simulink model "Single_Interlinking_Dual_Infinite_Bus_Window"  (R2024b)
settings: Solver=FixedStepAuto  StartTime=0  StopTime=35  FixedStep=Ts  RelTol=1e-3
InitFcn:
  | FS_Frequency=csvread("Frequency_Sweep_Log_Matched.csv",1,0);
values from neighbouring files (symbols this model uses):
  x_e = [i_d; i_q; i_d_i; i_q_i; v_d_i; v_q_i; theta; v_dc; v_dc_i; i; i_i; v_lk; p_sum_i; p_lk_i]    [InterlinkAcDcB2B.m]
undefined symbols (not defined in the file or in its folder): ApparatusDiscreDamping, ApparatusPara, ApparatusPowerFlow, ApparatusType, OtherInputs, PowerFlow, Ts, Wbase, Ybase, Zbase
libraries: SimplusGT x8, dspindex x4, spsControlledVoltageSourceLib x3, spsGroundLib x2, spsabctodq0Lib x2, spsThreePhaseSeriesRLCBranchLib x1, spsThreePhaseParallelRLCBranchLib x1, spsParallelRLCBranchLib x1, spsThreePhaseVIMeasurementLib x1, spsdq0toabcLib x1, sps_lib x1
settings Model: Creator=gzhan  LastModifiedBy=gzhan

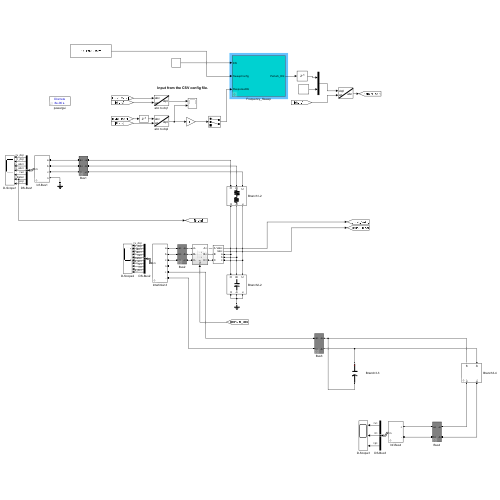
[thumbnail: Simulink's stored preview of the top-level diagram]
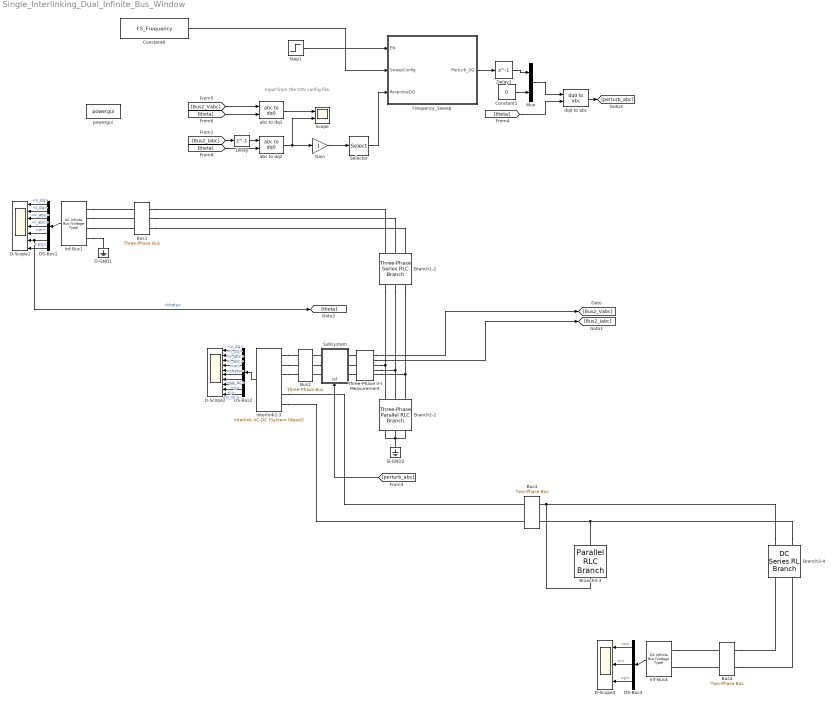
== system Single_Interlinking_Dual_Infinite_Bus_Window ==
  note: Input from the CSV config file.
  B-GND2 : spsGroundLib/Ground  LConnTagsString=a
  Branch1-2 : spsThreePhaseSeriesRLCBranchLib/Three-Phase Series RLC Branch  LConnTagsString=A|B|C  RConnTagsString=A|B|C  BranchType=RL  Resistance=(0.06)*Zbase  Inductance=(0.3)*Zbase/Wbase  Capacitance=1e-6  Measurements=None
  Branch2-2 : spsThreePhaseParallelRLCBranchLib/Three-Phase Parallel RLC Branch  LConnTagsString=A|B|C  RConnTagsString=A|B|C  BranchType=C  Resistance=(Inf)*Zbase  Inductance=(Inf)*Zbase/Wbase  Capacitance=(0.02)*Ybase/Wbase  Measurements=None
  Branch3-3 : spsParallelRLCBranchLib/Parallel RLC Branch  LConnTagsString=a  RConnTagsString=__new0  BranchType=C  Resistance=(Inf)*Zbase  Inductance=(Inf)*Zbase/Wbase  SetiL0=off  InitialCurrent=0  Capacitance=(0.02)*Ybase/Wbase  Setx0=off  InitialVoltage=0  Measurements=None
  Branch3-4 : SimplusGT/DC Series RL Branch  BranchType=RL  Resistance=(0.01)*Zbase  Inductance=(0.3)*Zbase/Wbase
      settings: SourceProductName=Simplus Grid Tool
  Bus1 : SimplusGT/Three-Phase Bus  Vbase=1  Sbase=1
      settings: SourceProductName=Simplus Grid Tool
  Bus2 : SimplusGT/Three-Phase Bus  Vbase=1  Sbase=1
      settings: SourceProductName=Simplus Grid Tool
  Bus3 : SimplusGT/Two-Phase Bus  Vbase=1  Sbase=1
      settings: SourceProductName=Simplus Grid Tool
  Bus4 : SimplusGT/Two-Phase Bus  Vbase=1  Sbase=1
      settings: SourceProductName=Simplus Grid Tool
  Constant1 : Constant  Value=0
  Constant8 : Constant  Value=FS_Frequency
  D-GND1 : spsGroundLib/Ground  LConnTagsString=a
  D-Scope1 : Scope  NumInputPorts=7
  D-Scope2 : Scope  NumInputPorts=10
  D-Scope3 : Scope  NumInputPorts=3
  DS-Bus1 : BusSelector  OutputSignals=v_dq,i_dq,v_abc,i_abc,w,theta,pq
  DS-Bus2 : BusSelector  OutputSignals=v_dq,i_dq,v_abc,i_abc,w,theta,pq_ac,v,i,p_dc
  DS-Bus3 : BusSelector  OutputSignals=v,i,p
  Delay : Delay  DelayLength=1
  Delay1 : Delay  DelayLength=1
  Frequency_Sweep : Subsystem  mask{Gain=0.1, Interval=1e-1}
      mask prompts: Gain "Output Gain"; Interval "Injection Interval"
  Gain : Gain  Gain=-1
  Inf-Bus1 : SimplusGT/AC Infinite Bus (Voltage Type)  Ts=Ts  Sbase=Sbase  Vbase=Vbase  Wbase=Wbase  vd=PowerFlow{1}(3)  vq=0  theta0=PowerFlow{1}(4)  w=Wbase  R=1e-30
      settings: SourceProductName=Simplus Grid Tool
  Inf-Bus4 : SimplusGT/DC Infinite Bus (Voltage Type)  Ts=Ts  Sbase=Sbase  Vbase=Vbase  v=PowerFlow{3}(3)  R=1e-30
      settings: SourceProductName=Simplus Grid Tool
  Interlink2-3 : SimplusGT/Interlink AC-DC (System Object)  Ts=Ts  Sbase=Sbase  Vbase=Vbase  Wbase=Wbase  ApparatusType=ApparatusType{2}  ApparatusPara=ApparatusPara{2}  PowerFlow=ApparatusPowerFlow{2}  x0=x_e{2}  OtherInputs=OtherInputs{2}  DiscreMethod=Hybrid Trapezoidal  EnableInsideModification=off  DiscreDampingFlag=on  DiscreDampingValue=ApparatusDiscreDamping{2}  LinearizationTimes=1  DirectFeedthrough=off
      settings: SourceProductName=Simplus Grid Tool
  Mux : Mux  Inputs=2
  Scope : Scope  NumInputPorts=2
  Selector : Selector  InputPortWidth=3  IndexOptions=Index vector (dialog)  Indices=[1 2]  OutputSizes=1
  Step1 : Step  Time=5  SampleTime=0
  Subsystem : Subsystem
      settings: PortSchema="{\"entries\":[{\"content\":{\"sides\":[{\"content\":{\"connectorIds\":[\"LConn1\",\"LConn2\",\"LConn3\"]},\"type\":\"ConnectorPlacement.EquallySpacedRectSide\",\"uuid\":\"320e3ad3-fe57-42ad-8679-028db54dd479\"},{\"content\":{\"connectorIds\":[\"RConn1\",\"RConn2\",\"RConn3\"],\"side\":\"RIGHT\"},\"type\":\"ConnectorPlacement.EquallySpacedRectSide\",\"uuid\":\"2b28e415-5225-4c3e-a28b-d8614ba274c6\"},{\"content\":{\"side\":\"TOP\"},\"type\":\"ConnectorPlacement.EquallySpacedRectSide\",\"uuid\":\"80974e19-6780-437b-9c92-3d578e35f276\"},{\"content\":{\"connectorIds\":[\"In1\"],\"side\":\"BOTTOM\"},\"type\":\"ConnectorPlacement.EquallySpacedRectSide\",\"uuid\":\"7f793f19-b02b-48c7-b373-3f4568a43fb5\"}]},\"type\":\"ConnectorPlacement.EquallySpacedConnector\",\"uuid\":\"fbbab89f-d0d6-4a2b-bd71-75cb5c2a328e\"}],\"packageUris\":[\"http://schema.mathworks.com/mf0/Connector/R2020b\"],\"version\":\"1.0\"}"
  Three-Phase V-I Measurement : spsThreePhaseVIMeasurementLib/Three-Phase V-I Measurement  VoltageMeasurement=phase-to-ground  SetLabelV=off  LabelV=Vabc  Vpu=off  VpuLL=off  CurrentMeasurement=yes  SetLabelI=off  LabelI=Iabc  Ipu=off  Pbase=100e6  Vbase=500e3  OutputType=Complex  PhasorSimulation=off  PSBequivalent=0
  abc to dq1 : spsabctodq0Lib/abc to dq0  Alignment=90 degrees behind phase A axis
  abc to dq2 : spsabctodq0Lib/abc to dq0  Alignment=90 degrees behind phase A axis
  dq0 to abc : spsdq0toabcLib/dq0 to abc  Alignment=90 degrees behind phase A axis
  powergui : sps_lib/powergui  Priority=1  SimulationMode=Discrete  SampleTime=Ts  frequency=60  Iterations=50  frequencyindice=0  Pbase=100e6  ErrMax=1e-4  UnitsV=kV  UnitsW=MW  buscounter=0  FunctionMessages=off  echomessages=off  EnableUseOfTLC=off  CurrentSourceSwitches=off  DisableSnubberDevices=off  DisableRonSwitches=off  DisableVfSwitches=off  DisplayEquations=off  AutomaticDiscreteSolvers=off  SolverType=Tustin/Backward Euler (TBE)  Interpol=off  ExternalGateDelay=off  methode=off  Ts=100  x0status=blocks  SPID=on  SwTol=0  HookPort=off  NonlinearTolerance=1e-4  nMaxIteration=100  ContinueOnMaxIteration=off  RestoreLinks=warning  ResistiveCurrentMeasurement=off  Frange=[0:2:500]  Ylog=off  Xlog=on  ShowGrid=off  save=off  variable=ZData  structure=0  ZoomFFT=off  StartTime=0.0  cycles=1  DisplayStyle=1  fundamental=60  FreqAxis=off  MaxFrequency=1000  frequencyindicesteady=1  RmsSteady=1  display=off
  wires:
  Inf-Bus1/1 -> DS-Bus1/1
  DS-Bus1/1 -> D-Scope1/1  "<v_dq>"
  DS-Bus1/2 -> D-Scope1/2  "<i_dq>"
  DS-Bus1/3 -> D-Scope1/3  "<v_abc>"
  DS-Bus1/4 -> D-Scope1/4  "<i_abc>"
  DS-Bus1/5 -> D-Scope1/5  "<w>"
  DS-Bus1/6 -> [theta], D-Scope1/6  "<theta>"
  DS-Bus1/7 -> D-Scope1/7  "<pq>"
  DS-Bus2/1 -> D-Scope2/1  "<v_dq>"
  DS-Bus2/2 -> D-Scope2/2  "<i_dq>"
  DS-Bus2/3 -> D-Scope2/3  "<v_abc>"
  DS-Bus2/4 -> D-Scope2/4  "<i_abc>"
  DS-Bus2/5 -> D-Scope2/5  "<w>"
  DS-Bus2/6 -> D-Scope2/6  "<theta>"
  DS-Bus2/7 -> D-Scope2/7  "<pq_ac>"
  DS-Bus2/8 -> D-Scope2/8  "<v>"
  DS-Bus2/9 -> D-Scope2/9  "<i>"
  DS-Bus2/10 -> D-Scope2/10  "<p_dc>"
  Inf-Bus4/1 -> DS-Bus3/1
  DS-Bus3/1 -> D-Scope3/1  "<v>"
  DS-Bus3/2 -> D-Scope3/2  "<i>"
  DS-Bus3/3 -> D-Scope3/3  "<p>"
  abc to dq1/1 -> Scope/1
  [theta] -> abc to dq1/2
  [Bus2_Iabc] -> Delay/1
  Gain/1 -> Selector/1
  Mux/1 -> dq0 to abc/1
  Step1/1 -> Frequency_Sweep/1(EN)
  [theta] -> abc to dq2/2
  Constant1/1 -> Mux/2
  [Bus2_Vabc] -> abc to dq1/1
  Delay/1 -> abc to dq2/1
  [theta] -> dq0 to abc/2
  Delay1/1 -> Mux/1
  abc to dq2/1 -> Scope/2, Gain/1
  Selector/1 -> Frequency_Sweep/3(ResponseDQ)
  Frequency_Sweep/1(Perturb_DQ) -> Delay1/1
  Constant8/1 -> Frequency_Sweep/2(SweepConfig)
  dq0 to abc/1 -> [perturb_abc]
  Three-Phase V-I Measurement/1 -> [Bus2_Vabc]
  [perturb_abc] -> Subsystem/1(ref)
  Three-Phase V-I Measurement/2 -> [Bus2_Iabc]
  Interlink2-3/1 -> DS-Bus2/1
  connections:
  Inf-Bus1/LConn4 -- D-GND1/LConn1
  Branch2-2/RConn1 -- Branch2-2/RConn2 -- Branch2-2/RConn3 -- B-GND2/LConn1
  Branch1-2/RConn1 -- Three-Phase V-I Measurement/RConn1 -- Branch2-2/LConn1
  Branch1-2/RConn2 -- Three-Phase V-I Measurement/RConn2 -- Branch2-2/LConn2
  Branch1-2/RConn3 -- Three-Phase V-I Measurement/RConn3 -- Branch2-2/LConn3
  Bus1/RConn1 -- Branch1-2/LConn1
  Bus1/RConn2 -- Branch1-2/LConn2
  Bus1/RConn3 -- Branch1-2/LConn3
  Bus4/RConn1 -- Branch3-4/RConn1
  Bus4/RConn2 -- Branch3-4/RConn2
  Branch3-4/LConn1 -- Bus3/RConn1 -- Branch3-3/RConn1
  Branch3-4/LConn2 -- Bus3/RConn2 -- Branch3-3/LConn1
  Inf-Bus1/LConn1 -- Bus1/LConn1
  Inf-Bus1/LConn2 -- Bus1/LConn2
  Inf-Bus1/LConn3 -- Bus1/LConn3
  Interlink2-3/LConn1 -- Bus2/LConn1
  Interlink2-3/LConn2 -- Bus2/LConn2
  Interlink2-3/LConn3 -- Bus2/LConn3
  Interlink2-3/LConn5 -- Bus3/LConn1
  Interlink2-3/LConn6 -- Bus3/LConn2
  Inf-Bus4/LConn1 -- Bus4/LConn1
  Inf-Bus4/LConn2 -- Bus4/LConn2
  Subsystem/LConn1 -- Bus2/RConn1
  Bus2/RConn2 -- Subsystem/LConn2
  Subsystem/LConn3 -- Bus2/RConn3
  Subsystem/RConn1 -- Three-Phase V-I Measurement/LConn1
  Three-Phase V-I Measurement/LConn2 -- Subsystem/RConn2
  Subsystem/RConn3 -- Three-Phase V-I Measurement/LConn3

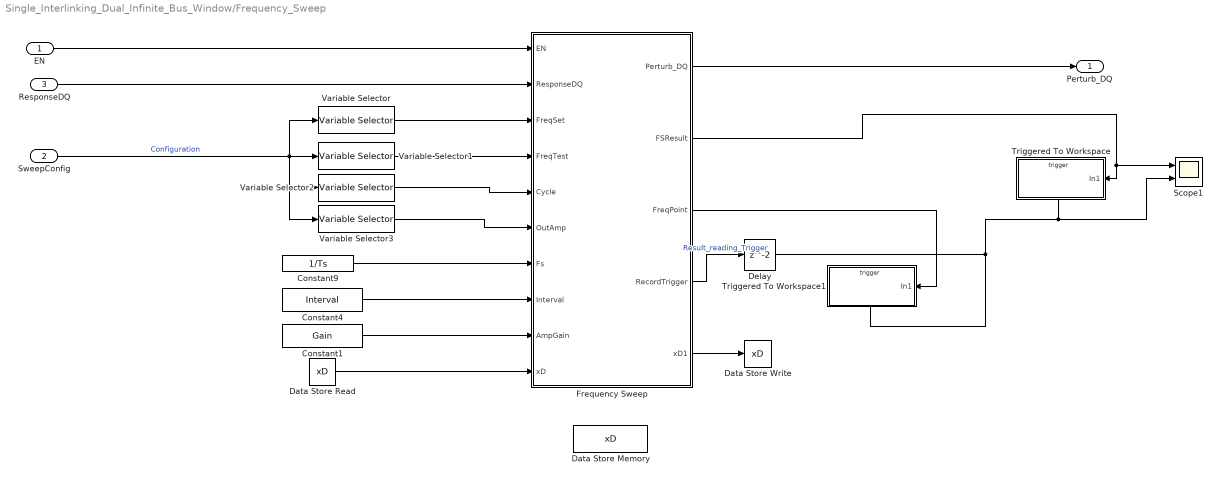
== system Single_Interlinking_Dual_Infinite_Bus_Window/Frequency_Sweep ==
  EN : Inport
  SweepConfig : Inport  Port=2
  ResponseDQ : Inport  Port=3
  Constant1 : Constant  Value=Gain
  Constant4 : Constant  Value=Interval
  Constant9 : Constant  Value=1/Ts
  Data Store Memory : DataStoreMemory  DataStoreName=xD  WriteAfterWriteMsg=warning  InitialValue=zeros(1,18)  ShowAdditionalParam=off
  Data Store Read : DataStoreRead  DataStoreName=xD  IndexOptions=Index vector (dialog)  Indices=1  OutputSizes=1
  Data Store Write : DataStoreWrite  DataStoreName=xD  IndexOptions=Index vector (dialog)  Indices=1  OutputSizes=1
  Delay : Delay
  Frequency Sweep : MATLAB Function  TreatAsAtomicUnit=on
  Scope1 : Scope  NumInputPorts=2
  Triggered To Workspace : Subsystem  AncestorBlock=dspsnks4/Triggered To Workspace  TreatAsAtomicUnit=on  mask(Triggered To Workspace){TriggerType=Rising edge, VariableName=FS_Result, Buffer=5000, Decimation=1, Save2DMode=2-D array (concatenate along first dimension), FixptAsFi=off}
      mask prompts: TriggerType "dsp:TriggeredToWorkspaceBlockDialog:TriggerType_MP"; VariableName "dsp:TriggeredToWorkspaceBlockDialog:VariableName_MP"; Buffer "dsp:TriggeredToWorkspaceBlockDialog:Buffer_MP"; Decimation "dsp:TriggeredToWorkspaceBlockDialog:Decimation_MP"; Save2DMode "dsp:TriggeredToWorkspaceBlockDialog:Save2DMode_MP"; FixptAsFi "dsp:TriggeredToWorkspaceBlockDialog:FixptAsFi_MP"
      mask help: dsp:TriggeredToWorkspaceBlockDialog:TriggeredToWorkspace_MaskDesc
      mask init:
      | dspblktrigtwks('init',TriggerType);
      settings: CopyFcn=dspblkcopystw(gcbh);
      mask Help: eval('blocksethelp');
      mask TypeOptions TriggerType: dsp:TriggeredToWorkspaceBlockDialog:TriggerType_RisingEdge | dsp:TriggeredToWorkspaceBlockDialog:TriggerType_FallingEdge | dsp:TriggeredToWorkspaceBlockDialog:TriggerType_EitherEdge
      mask TypeOptions Save2DMode: dsp:TriggeredToWorkspaceBlockDialog:Save2DMode_2DArray | dsp:TriggeredToWorkspaceBlockDialog:Save2DMode_3DArray
      mask DialogControl TriggerType Prompt: Trigger type:
      mask DialogControl VariableName Prompt: Variable name:
      mask DialogControl Buffer Prompt: Maximum number of rows:
      mask DialogControl Decimation Prompt: Decimation:
      mask DialogControl Save2DMode Prompt: Save 2-D signals as:
      mask DialogControl FixptAsFi Prompt: Log fixed-point data as a fi object
      mask Display: disp(get_param(gcbh,'VariableName'))
  Triggered To Workspace1 : Subsystem  AncestorBlock=dspsnks4/Triggered To Workspace  TreatAsAtomicUnit=on  mask(Triggered To Workspace){TriggerType=Rising edge, VariableName=FS_Freq_point, Buffer=5000, Decimation=1, Save2DMode=2-D array (concatenate along first dimension), FixptAsFi=off}
      mask prompts: TriggerType "dsp:TriggeredToWorkspaceBlockDialog:TriggerType_MP"; VariableName "dsp:TriggeredToWorkspaceBlockDialog:VariableName_MP"; Buffer "dsp:TriggeredToWorkspaceBlockDialog:Buffer_MP"; Decimation "dsp:TriggeredToWorkspaceBlockDialog:Decimation_MP"; Save2DMode "dsp:TriggeredToWorkspaceBlockDialog:Save2DMode_MP"; FixptAsFi "dsp:TriggeredToWorkspaceBlockDialog:FixptAsFi_MP"
      mask help: dsp:TriggeredToWorkspaceBlockDialog:TriggeredToWorkspace_MaskDesc
      mask init:
      | dspblktrigtwks('init',TriggerType);
      settings: CopyFcn=dspblkcopystw(gcbh);
      mask Help: eval('blocksethelp');
      mask TypeOptions TriggerType: dsp:TriggeredToWorkspaceBlockDialog:TriggerType_RisingEdge | dsp:TriggeredToWorkspaceBlockDialog:TriggerType_FallingEdge | dsp:TriggeredToWorkspaceBlockDialog:TriggerType_EitherEdge
      mask TypeOptions Save2DMode: dsp:TriggeredToWorkspaceBlockDialog:Save2DMode_2DArray | dsp:TriggeredToWorkspaceBlockDialog:Save2DMode_3DArray
      mask DialogControl TriggerType Prompt: Trigger type:
      mask DialogControl VariableName Prompt: Variable name:
      mask DialogControl Buffer Prompt: Maximum number of rows:
      mask DialogControl Decimation Prompt: Decimation:
      mask DialogControl Save2DMode Prompt: Save 2-D signals as:
      mask DialogControl FixptAsFi Prompt: Log fixed-point data as a fi object
      mask Display: disp(get_param(gcbh,'VariableName'))
  Variable Selector : dspindex/Variable Selector  NumInputs=1  rowsOrCols=Columns  IdxMode=Fixed  Elements=1  ZerOneIdxMode=One-based  errmode=Clip Index  FillMode=on  FillValues=0
  Variable Selector1 : dspindex/Variable Selector  NumInputs=1  rowsOrCols=Columns  IdxMode=Fixed  Elements=2  ZerOneIdxMode=One-based  errmode=Clip Index  FillMode=on  FillValues=0
  Variable Selector2 : dspindex/Variable Selector  NumInputs=1  rowsOrCols=Columns  IdxMode=Fixed  Elements=3  ZerOneIdxMode=One-based  errmode=Clip Index  FillMode=on  FillValues=0
  Variable Selector3 : dspindex/Variable Selector  NumInputs=1  rowsOrCols=Columns  IdxMode=Fixed  Elements=4  ZerOneIdxMode=One-based  errmode=Clip Index  FillMode=on  FillValues=0
  Perturb_DQ : Outport
  wires:
  Variable Selector2/1 -> Frequency Sweep/5(Cycle)
  Frequency Sweep/2(FSResult) -> Triggered To Workspace/1(In1), Scope1/1
  Frequency Sweep/4(RecordTrigger) -> Delay/1  "Result_reading_Trigger"
  Constant4/1 -> Frequency Sweep/8(Interval)
  Frequency Sweep/5(xD1) -> Data Store Write/1
  Variable Selector3/1 -> Frequency Sweep/6(OutAmp)
  Variable Selector1/1 -> Frequency Sweep/4(FreqTest)
  SweepConfig/1 -> Variable Selector3/1, Variable Selector2/1, Variable Selector1/1, Variable Selector/1  "Configuration"
  ResponseDQ/1 -> Frequency Sweep/2(ResponseDQ)
  Variable Selector/1 -> Frequency Sweep/3(FreqSet)
  Frequency Sweep/3(FreqPoint) -> Triggered To Workspace1/1(In1)
  Data Store Read/1 -> Frequency Sweep/10(xD)
  Constant9/1 -> Frequency Sweep/7(Fs)
  Frequency Sweep/1(Perturb_DQ) -> Perturb_DQ/1
  EN/1 -> Frequency Sweep/1(EN)
  Delay/1 -> Scope1/2, Triggered To Workspace/Trigger, Triggered To Workspace1/Trigger
  Constant1/1 -> Frequency Sweep/9(AmpGain)

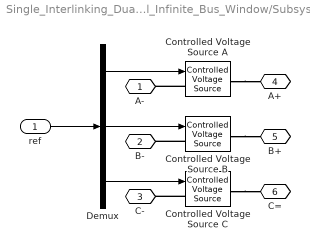
== system Single_Interlinking_Dual_Infinite_Bus_Window/Subsystem ==
  ref : Inport
  Controlled Voltage Source A : spsControlledVoltageSourceLib/Controlled Voltage Source  Initialize=on  Source_Type=AC  Amplitude=0  Phase=0  Frequency=0  Measurements=None
  Controlled Voltage Source B : spsControlledVoltageSourceLib/Controlled Voltage Source  Initialize=on  Source_Type=AC  Amplitude=0  Phase=0  Frequency=0  Measurements=None
  Controlled Voltage Source C : spsControlledVoltageSourceLib/Controlled Voltage Source  Initialize=on  Source_Type=AC  Amplitude=0  Phase=0  Frequency=0  Measurements=None
  Demux : Demux  Outputs=3
  A- : PMIOPort  Side=Left
  B- : PMIOPort  Port=2  Side=Left
  C- : PMIOPort  Port=3  Side=Left
  A+ : PMIOPort  Port=4  Side=Right
  B+ : PMIOPort  Port=5  Side=Right
  C= : PMIOPort  Port=6  Side=Right
  wires:
  Demux/3 -> Controlled Voltage Source C/1
  Demux/2 -> Controlled Voltage Source B/1
  Demux/1 -> Controlled Voltage Source A/1
  ref/1 -> Demux/1
  connections:
  Controlled Voltage Source C/RConn1 -- C=/RConn1
  Controlled Voltage Source C/LConn1 -- C-/RConn1
  Controlled Voltage Source A/LConn1 -- A-/RConn1
  Controlled Voltage Source B/LConn1 -- B-/RConn1
  Controlled Voltage Source A/RConn1 -- A+/RConn1
  Controlled Voltage Source B/RConn1 -- B+/RConn1

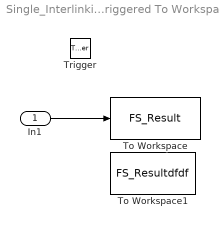
== system Single_Interlinking_Dual_Infinite_Bus_Window/Frequency_Sweep/Triggered To Workspace ==
  In1 : Inport
  Trigger : TriggerPort  VariantControl=Variant
  To Workspace : ToWorkspace  VariableName=FS_Result  SampleTime=-1
      settings: Save2DSignal=2-D array (concatenate along first dimension)
  To Workspace1 : ToWorkspace  VariableName=FS_Resultdfdf  SampleTime=-1
      settings: Save2DSignal=2-D array (concatenate along first dimension)
  wires:
  In1/1 -> To Workspace/1

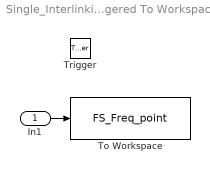
== system Single_Interlinking_Dual_Infinite_Bus_Window/Frequency_Sweep/Triggered To Workspace1 ==
  In1 : Inport
  Trigger : TriggerPort  VariantControl=Variant
  To Workspace : ToWorkspace  VariableName=FS_Freq_point  SampleTime=-1
      settings: Save2DSignal=2-D array (concatenate along first dimension)
  wires:
  In1/1 -> To Workspace/1

== matlab function Single_Interlinking_Dual_Infinite_Bus_Window/Frequency_Sweep/Frequency Sweep ==
  data: EN input; Perturb_DQ output; ResponseDQ input size=[1 2]; FreqSet input; FreqTest input; Cycle input; OutAmp input; Fs input; Interval input; AmpGain input; xD input; FSResult output; FreqPoint output; RecordTrigger output; xD1 output
function [Perturb_DQ, FSResult, FreqPoint, RecordTrigger, xD1] = fcn(EN,ResponseDQ, FreqSet, FreqTest, Cycle, OutAmp, Fs, Interval, AmpGain, xD)
% Real-time frequency scanning with Hann window + DC detrend (running mean)
%
% State variables (xD):
% xD1:  case (CaseK)
% xD2:  Ns  (total time steps for output at current frequency)
% xD3:  Nt  (total time steps for test frequency integration)
% xD4:  n   (sample count in current segment, starts at 1)
% xD5:  kc  (frequency index)
% xD6:  OutD
% xD7:  OutQ
% xD8:  SumDRe
% xD9:  SumDIm
% xD10: SumQRe
% xD11: SumQIm
% xD12: FinalDRe
% xD13: FinalDIm
% xD14: FinalQRe
% xD15: FinalQIm
% xD16: TWait
% xD17: MeanD   (running mean of ResponseDQ(1))   <-- NEW
% xD18: MeanQ   (running mean of ResponseDQ(2))   <-- NEW

% --- read states
CaseK   = xD(1);
Ns      = xD(2);
Nt      = xD(3);
n       = xD(4);
kc      = xD(5);
OutD    = xD(6);
OutQ    = xD(7);
SumDRe  = xD(8);
SumDIm  = xD(9);
SumQRe  = xD(10);
SumQIm  = xD(11);
FinalDRe= xD(12);
FinalDIm= xD(13);
FinalQRe= xD(14);
FinalQIm= xD(15);
TWait   = xD(16);
MeanD   = xD(17);   % NEW
MeanQ   = xD(18);   % NEW

FrequencyNum = length(FreqSet);

if AmpGain==0
    error('gain must not be zero');
end

%% Main Loop
if EN==0   % if Enable 0, reset just outputs (keep states unless you want full reset)
    OutD = 0;
    OutQ = 0;
else
    switch CaseK
        case 0 % the very first round
            kc    = 1;
            CaseK = 1;

        case 1 % set up D-axis sweep for this frequency index
            if kc>FrequencyNum         % sweep finished. Go to case 9
                OutD = 0;
                OutQ = 0;
                CaseK = 9;
            elseif Cycle(kc)==0        % skip this frequency
                kc = kc + 1;
            else
                % reset integrators and counters
                SumDRe = 0; SumDIm = 0; SumQRe = 0; SumQIm = 0;
                TWait  = 0; n = 0;
                MeanD  = 0; MeanQ  = 0;   % NEW: reset running means

                % total time steps for this frequency
                Ns = Fs/FreqSet(kc)*Cycle(kc); % for output count
                Nt = Fs/FreqTest(kc)*Cycle(kc); % for frequency test count

                % prime first output sample (n will become 1)
                OutD = OutAmp(kc)*sin(2*pi*Cycle(kc)*n/Ns)*AmpGain;
                OutQ = 0;
                n    = n + 1;
                CaseK= 2;
            end

        case 2 % sweep D axis: inject D, demod both D/Q responses
            OutD = OutAmp(kc)*sin(2*pi*Cycle(kc)*n/Ns)*AmpGain;
            OutQ = 0;

            % --- Hann window (periodic) at this sample (n in 1..Nt)
            w  = 0.5 - 0.5*cos(2*pi*(n-1)/Nt);

            % --- update online running means for DC detrend
            MeanD = MeanD + (ResponseDQ(1) - MeanD)/n;
            MeanQ = MeanQ + (ResponseDQ(2) - MeanQ)/n;

            % --- detrended, windowed samples
            yD = (ResponseDQ(1) - MeanD) * w;
            yQ = (ResponseDQ(2) - MeanQ) * w;

            % --- demodulate at test frequency
            sn = sin(2*pi*Cycle(kc)*(n-1)/Nt);
            cn = cos(2*pi*Cycle(kc)*(n-1)/Nt);

            % Accumulate (real=sin, imag=cos; sign convention consistent)
            SumDRe = SumDRe + yD * sn;
            SumDIm = SumDIm + yD * cn;
            SumQRe = SumQRe + yQ * sn;
            SumQIm = SumQIm + yQ * cn;

            if (n<Nt)
                n = n + 1;
            else
                OutD = 0;
                OutQ = 0;
                CaseK= 3;
            end

        case 3 % finalize D-axis phasor; wait (settling) before Q sweep
            % Hann coherent gain
            cg = 0.5;

            % Normalization (kept your original form, divided by cg)
            FinalDRe = (2*SumDRe*FreqSet(kc)/Cycle(kc)/Fs/OutAmp(kc)/AmpGain)/cg;
            FinalDIm = (2*SumDIm*FreqSet(kc)/Cycle(kc)/Fs/OutAmp(kc)/AmpGain)/cg;
            FinalQRe = (2*SumQRe*FreqSet(kc)/Cycle(kc)/Fs/OutAmp(kc)/AmpGain)/cg;
            FinalQIm = (2*SumQIm*FreqSet(kc)/Cycle(kc)/Fs/OutAmp(kc)/AmpGain)/cg;

            if TWait<Fs*Interval
                TWait = TWait + 1;
            else
                TWait = 0;
                CaseK = 4;
            end

        case 4 % prepare Q-axis sweep
            SumDRe = 0; SumDIm = 0; SumQRe = 0; SumQIm = 0;
            TWait  = 0; n = 0;
            MeanD  = 0; MeanQ  = 0;   % NEW: reset running means

            % total time steps for this frequency
            Ns = Fs/FreqSet(kc)*Cycle(kc); % for output count
            Nt = Fs/FreqTest(kc)*Cycle(kc); % for frequency test count

            OutD = 0;
            OutQ = OutAmp(kc)*sin(2*pi*Cycle(kc)*n/Ns)*AmpGain;
            n    = n + 1;
            CaseK= 5;

        case 5 % sweep Q axis: inject Q, demod both D/Q responses
            OutD = 0;
            OutQ = OutAmp(kc)*sin(2*pi*Cycle(kc)*n/Ns)*AmpGain;

            % --- Hann window (periodic)
            w  = 0.5 - 0.5*cos(2*pi*(n-1)/Nt);

            % --- running means
            MeanD = MeanD + (ResponseDQ(1) - MeanD)/n;
            MeanQ = MeanQ + (ResponseDQ(2) - MeanQ)/n;

            % --- detrended, windowed
            yD = (ResponseDQ(1) - MeanD) * w;
            yQ = (ResponseDQ(2) - MeanQ) * w;

            % --- demodulate
            sn = sin(2*pi*Cycle(kc)*(n-1)/Nt);
            cn = cos(2*pi*Cycle(kc)*(n-1)/Nt);

            % Accumulate
            SumDRe = SumDRe + yD * sn;
            SumDIm = SumDIm + yD * cn;
            SumQRe = SumQRe + yQ * sn;
            SumQIm = SumQIm + yQ * cn;

            if (n<Nt)
                n = n + 1;
            else
                OutD = 0;
                OutQ = 0;
                CaseK= 6;
            end

        case 6 % finalize Q-axis phasor; advance to next frequency
            cg = 0.5; % Hann coherent gain

            FinalDRe = (2*SumDRe*FreqSet(kc)/Cycle(kc)/Fs/OutAmp(kc)/AmpGain)/cg;
            FinalDIm = (2*SumDIm*FreqSet(kc)/Cycle(kc)/Fs/OutAmp(kc)/AmpGain)/cg;
            FinalQRe = (2*SumQRe*FreqSet(kc)/Cycle(kc)/Fs/OutAmp(kc)/AmpGain)/cg;
            FinalQIm = (2*SumQIm*FreqSet(kc)/Cycle(kc)/Fs/OutAmp(kc)/AmpGain)/cg;

            if TWait<Fs*Interval
                TWait = TWait + 1;
            else
                TWait = 0;
                kc    = kc + 1;
                CaseK = 1;
            end

        case 9 % finished; outputs zero
            % nothing
    end
end

%% set outputs/state
xD1 = [CaseK,Ns,Nt,n,kc,OutD,OutQ,SumDRe,SumDIm,SumQRe,SumQIm,FinalDRe,FinalDIm,FinalQRe,FinalQIm,TWait,MeanD,MeanQ];
Perturb_DQ = [OutD,OutQ];

if kc>0 && EN==1
    FSResult = [FinalDRe+1i*FinalDIm, FinalQRe+1i*FinalQIm]; % complex result
    if kc>FrequencyNum
        kc = FrequencyNum;
    end
    FreqPoint = FreqSet(kc);
else
    FSResult  = [0,0];
    FreqPoint = 0;
end

% Trigger: after each axis completes (aligned with your original intent)
if CaseK==3 || CaseK==6
    RecordTrigger = 1;
else
    RecordTrigger = 0;
end

end
